simulink model "Table_de_mixage"  (R2020a)
settings: Solver=VariableStepAuto  StartTime=0.0  StopTime=10.0  RelTol=1e-3
undefined symbols (not defined in the file): fdesignblkfcn, gcbh
libraries: dspspect3 x3, dsparch4 x1, dspsrcs4 x1, dspvision x1, dspobslib x1, simulink x1
settings Model: Creator=XPS 15  LastModifiedBy=XPS 15

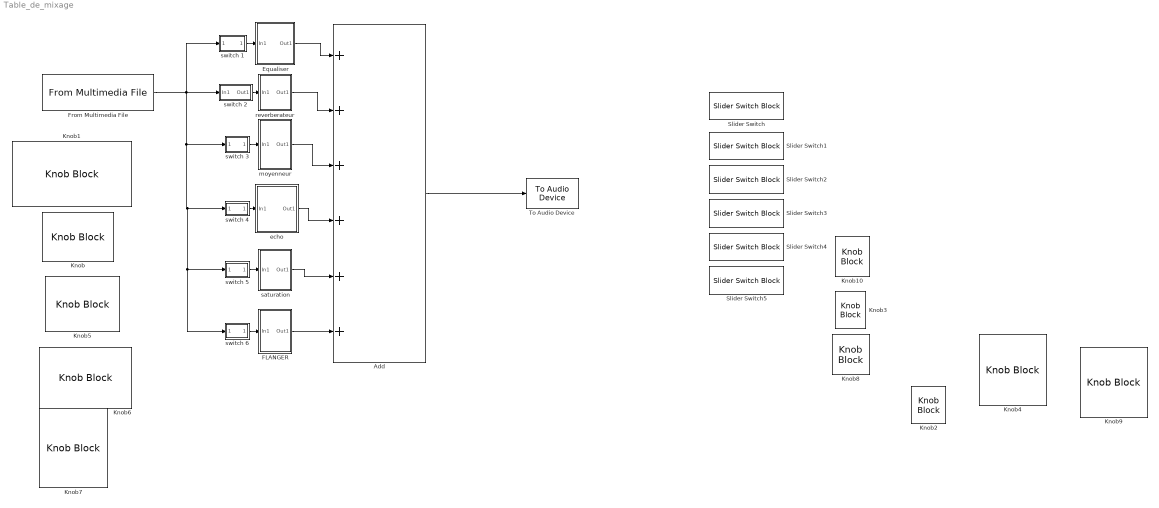
== system Table_de_mixage ==
  Add : Sum  Inputs=++++++
  Equaliser : Subsystem
  FLANGER : Subsystem
  From Multimedia File : dspvision/From Multimedia File  inputFilename=C:\Users\XPS 15\Desktop\L05 Sorbonne\images\Son\Projet\guitare.wav  readRange=[1 Inf]  loop=on  numPlays=inf  outputStreams=Audio only  videoDataType=single  audioDataType=double  inheritSampleTime=on  userDefinedSampleTime=1/30  noAudioOutput=off  isIntensityVideo=off  fourcc=RGB  colorVideoFormat=Separate color signals  outputEOF=off  dataOrg=Column-major  audioFrameSize=11025  computeAudioFrameSize=off  outSamplingMode=Sample based
  Knob{,1,3,5..8,10} (8 alike) : KnobBlock  ScaleMax=1
  Knob2 : KnobBlock
  Knob4 : KnobBlock
  Knob9 : KnobBlock
  Slider Switch{,1..5} (6 alike) : SliderSwitchBlock
      settings: Values={{'Off', 'On'}, [0 1]}
  To Audio Device : dspobslib/To Audio Device  deviceName=Default  inheritSampleRate=on  sampleRate=44100  deviceDatatype=Determine from input data type  autoBufferSize=on  bufferSize=4096  queueDuration=1.0  defaultOutputChannelMapping=on  outputChannelMapping=1:2  outputNumUnderrunSamples=off
      settings: SourceProductBaseCode=DS
  echo : Subsystem
  moyenneur : Subsystem
  reverberateur : Subsystem
  saturation : Subsystem
  switch 1 : Subsystem
  switch 2 : Subsystem
  switch 3 : Subsystem
  switch 4 : Subsystem
  switch 5 : Subsystem
  switch 6 : Subsystem
  wires:
  Equaliser/1(Out1) -> Add/1
  saturation/1(Out1) -> Add/5
  echo/1(Out1) -> Add/4
  moyenneur/1(Out1) -> Add/3
  reverberateur/1(Out1) -> Add/2
  switch 1/1(Out1) -> Equaliser/1(In1)
  From Multimedia File/1 -> switch 6/1(In1), switch 5/1(In1), switch 4/1(In1), switch 3/1(In1), switch 2/1(In1), switch 1/1(In1)
  switch 2/1(Out1) -> reverberateur/1(In1)
  switch 3/1(Out1) -> moyenneur/1(In1)
  switch 4/1(Out1) -> echo/1(In1)
  switch 5/1(Out1) -> saturation/1(In1)
  FLANGER/1(Out1) -> Add/6
  switch 6/1(Out1) -> FLANGER/1(In1)
  Add/1 -> To Audio Device/1

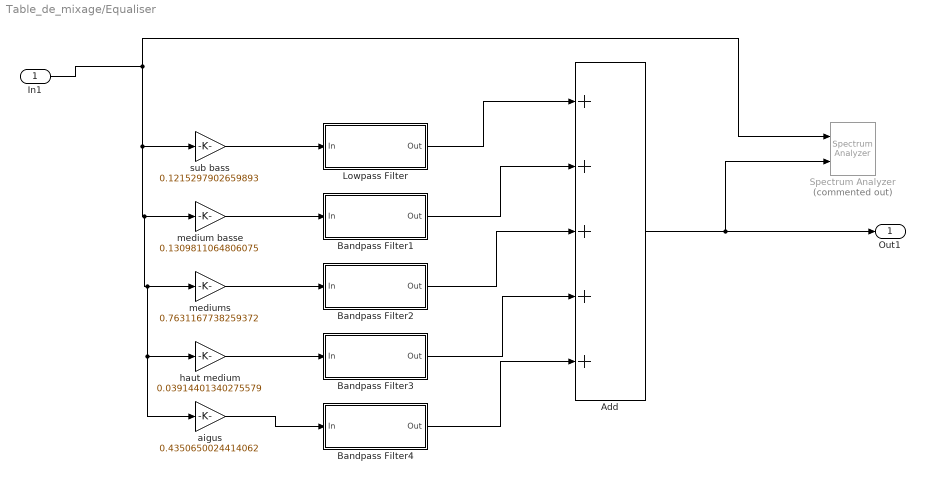
== system Table_de_mixage/Equaliser ==
  In1 : Inport
  Add : Sum  Inputs=+++++
  Bandpass Filter1 : Subsystem  DialogController=fdesignblkfcn  InitFcn=fdesignblkfcn(gcbh, {'InitFcn'});  mask(Bandpass Filter){}
      mask help: Design a bandpass filter
      settings: CopyFcn=fdesignblkfcn(gcbh, {'CopyFcn'});
      mask Help: helpview(mapfilelocation('dsp'), 'dspbandpassfilter');
      mask Display: disp('Bandpass');
  Bandpass Filter2 : Subsystem  DialogController=fdesignblkfcn  InitFcn=fdesignblkfcn(gcbh, {'InitFcn'});  mask(Bandpass Filter){}
      mask help: Design a bandpass filter
      settings: CopyFcn=fdesignblkfcn(gcbh, {'CopyFcn'});
      mask Help: helpview(mapfilelocation('dsp'), 'dspbandpassfilter');
      mask Display: disp('Bandpass');
  Bandpass Filter3 : Subsystem  DialogController=fdesignblkfcn  InitFcn=fdesignblkfcn(gcbh, {'InitFcn'});  mask(Bandpass Filter){}
      mask help: Design a bandpass filter
      settings: CopyFcn=fdesignblkfcn(gcbh, {'CopyFcn'});
      mask Help: helpview(mapfilelocation('dsp'), 'dspbandpassfilter');
      mask Display: disp('Bandpass');
  Bandpass Filter4 : Subsystem  DialogController=fdesignblkfcn  InitFcn=fdesignblkfcn(gcbh, {'InitFcn'});  mask(Bandpass Filter){}
      mask help: Design a bandpass filter
      settings: CopyFcn=fdesignblkfcn(gcbh, {'CopyFcn'});
      mask Help: helpview(mapfilelocation('dsp'), 'dspbandpassfilter');
      mask Display: disp('Bandpass');
  Lowpass Filter : Subsystem  DialogController=fdesignblkfcn  InitFcn=fdesignblkfcn(gcbh, {'InitFcn'});  mask(Lowpass Filter){}
      mask help: Design a lowpass filter
      settings: CopyFcn=fdesignblkfcn(gcbh, {'CopyFcn'});
      mask Help: helpview(mapfilelocation('dsp'), 'dsplowpassfilter');
      mask Display: disp('Lowpass')
  Spectrum Analyzer : SpectrumAnalyzer  Commented=on  NumInputPorts=2
  aigus : Gain  Gain=0.4350650024414062
  haut medium : Gain  Gain=0.03914401340275579
  medium basse : Gain  Gain=0.1309811064806075
  mediums : Gain  Gain=0.7631167738259372
  sub bass : Gain  Gain=0.1215297902659893
  Out1 : Outport
  wires:
  Lowpass Filter/1(Out) -> Add/1
  haut medium/1 -> Bandpass Filter3/1(In)
  sub bass/1 -> Lowpass Filter/1(In)
  In1/1 -> aigus/1, haut medium/1, mediums/1, medium basse/1, sub bass/1, Spectrum Analyzer/1
  mediums/1 -> Bandpass Filter2/1(In)
  Bandpass Filter3/1(Out) -> Add/4
  Add/1 -> Out1/1, Spectrum Analyzer/2
  medium basse/1 -> Bandpass Filter1/1(In)
  Bandpass Filter2/1(Out) -> Add/3
  Bandpass Filter4/1(Out) -> Add/5
  aigus/1 -> Bandpass Filter4/1(In)
  Bandpass Filter1/1(Out) -> Add/2

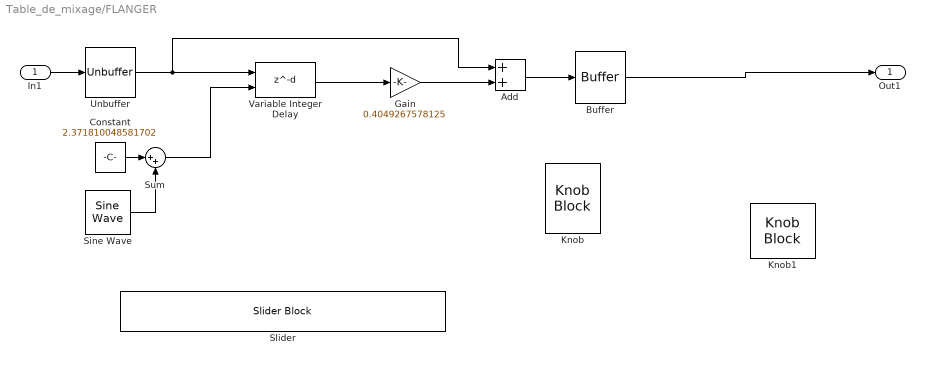
== system Table_de_mixage/FLANGER ==
  In1 : Inport
  Add : Sum
  Buffer : Buffer  N=11025  OutputFrames=off
  Constant : Constant  Value=2.371810048581702
  Gain : Gain  Gain=0.4049267578125
  Knob : KnobBlock  ScaleMax=5
  Knob1 : KnobBlock  ScaleMax=1
  Sine Wave : dspsrcs4/Sine Wave  Amplitude=1  Frequency=804.9368351063829  Phase=0  SampleMode=Discrete  OutComplex=Real  CompMethod=Trigonometric fcn  TableSize=Speed  SampleTime=1/11025  SamplesPerFrame=1  ResetState=Restart at time zero  OutputFrames=off  dataType=double  wordLen=16  udDataType=sfix(16)  fracBitsMode=Best precision  numFracBits=15  OutDataTypeStr=double  LastOutDataTypeStr=double
  Slider : SliderBlock  ScaleMax=10000
  Sum : Sum  Inputs=|++
  Unbuffer : Unbuffer
  Variable Integer Delay : Delay  DelayLengthSource=Input port
      settings: InputPortMap=u0,p1
  Out1 : Outport
  wires:
  In1/1 -> Unbuffer/1
  Unbuffer/1 -> Add/1, Variable Integer Delay/1
  Constant/1 -> Sum/1
  Sine Wave/1 -> Sum/2
  Sum/1 -> Variable Integer Delay/2
  Variable Integer Delay/1 -> Gain/1
  Gain/1 -> Add/2
  Add/1 -> Buffer/1
  Buffer/1 -> Out1/1

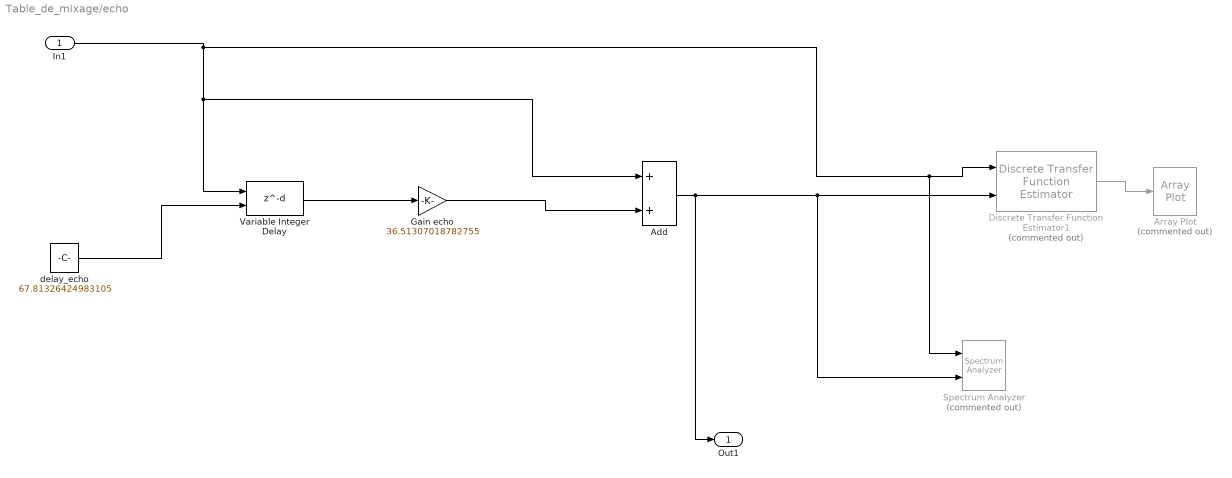
== system Table_de_mixage/echo ==
  In1 : Inport
  Add : Sum
  Array Plot : ArrayPlot  Commented=on
  Discrete Transfer Function Estimator1 : dspspect3/Discrete Transfer Function Estimator  Commented=on  WindowMode=Specify on dialog  WindowLength=1024  Overlap=50  AveragingMethod=Running  ForgettingFactorPort=off  ForgettingFactor=0.9  SpectralAverages=100  FFTLengthSource=Auto  FFTLength=128  Window=Hann  SidelobeAttenuation=60  FrequencyRange=One-sided  OutputCoherence=off  SimulateUsing=Code generation
      settings: SourceProductBaseCode=DS
  Gain echo : Gain  Gain=36.51307018782755
  Spectrum Analyzer : SpectrumAnalyzer  Commented=on  NumInputPorts=2
  Variable Integer Delay : Delay  DelayLengthSource=Input port
      settings: InputPortMap=u0,p1
  delay_echo : Constant  Value=67.81326424983105
  Out1 : Outport
  wires:
  Add/1 -> Discrete Transfer Function Estimator1/2, Spectrum Analyzer/2, Out1/1
  Variable Integer Delay/1 -> Gain echo/1
  In1/1 -> Variable Integer Delay/1, Add/1, Spectrum Analyzer/1, Discrete Transfer Function Estimator1/1
  Gain echo/1 -> Add/2
  Discrete Transfer Function Estimator1/1 -> Array Plot/1
  delay_echo/1 -> Variable Integer Delay/2

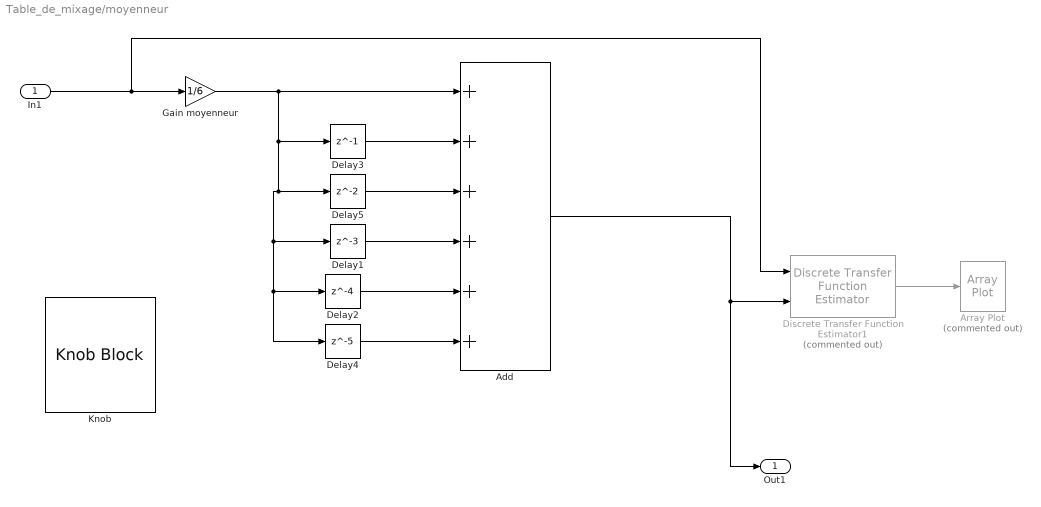
== system Table_de_mixage/moyenneur ==
  In1 : Inport
  Add : Sum  Inputs=++++++
  Array Plot : ArrayPlot  Commented=on
  Delay1 : Delay  DelayLength=3  InitialCondition=0  InputProcessing=Columns as channels (frame based)
  Delay2 : Delay  DelayLength=4  InitialCondition=0  InputProcessing=Columns as channels (frame based)
  Delay3 : Delay  DelayLength=1  InitialCondition=0  InputProcessing=Columns as channels (frame based)
  Delay4 : Delay  DelayLength=5  InitialCondition=0  InputProcessing=Columns as channels (frame based)
  Delay5 : Delay  InitialCondition=0  InputProcessing=Columns as channels (frame based)
  Discrete Transfer Function Estimator1 : dspspect3/Discrete Transfer Function Estimator  Commented=on  WindowMode=Specify on dialog  WindowLength=1024  Overlap=50  AveragingMethod=Running  ForgettingFactorPort=off  ForgettingFactor=0.9  SpectralAverages=100  FFTLengthSource=Auto  FFTLength=128  Window=Hann  SidelobeAttenuation=60  FrequencyRange=One-sided  OutputCoherence=off  SimulateUsing=Code generation
      settings: SourceProductBaseCode=DS
  Gain moyenneur : Gain  Gain=1/6
  Knob : KnobBlock
  Out1 : Outport
  wires:
  Delay4/1 -> Add/6
  Delay5/1 -> Add/3
  Gain moyenneur/1 -> Delay5/1, Delay1/1, Delay2/1, Delay4/1, Delay3/1, Add/1
  Discrete Transfer Function Estimator1/1 -> Array Plot/1
  Delay1/1 -> Add/4
  Add/1 -> Out1/1, Discrete Transfer Function Estimator1/2
  Delay2/1 -> Add/5
  In1/1 -> Discrete Transfer Function Estimator1/1, Gain moyenneur/1
  Delay3/1 -> Add/2

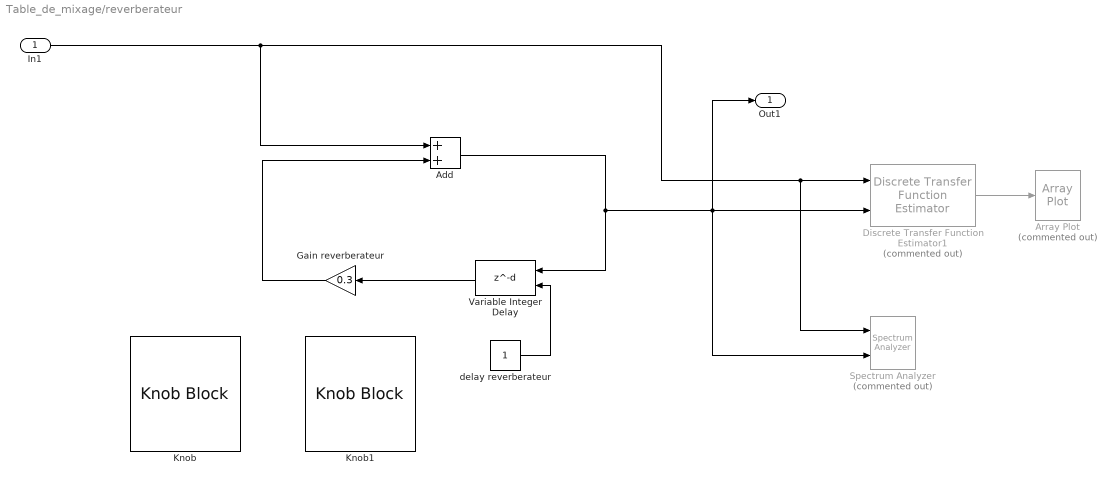
== system Table_de_mixage/reverberateur ==
  In1 : Inport
  Add : Sum
  Array Plot : ArrayPlot  Commented=on
  Discrete Transfer Function Estimator1 : dspspect3/Discrete Transfer Function Estimator  Commented=on  WindowMode=Specify on dialog  WindowLength=1024  Overlap=50  AveragingMethod=Running  ForgettingFactorPort=off  ForgettingFactor=0.9  SpectralAverages=100  FFTLengthSource=Auto  FFTLength=128  Window=Hann  SidelobeAttenuation=60  FrequencyRange=One-sided  OutputCoherence=off  SimulateUsing=Code generation
      settings: SourceProductBaseCode=DS
  Gain reverberateur : Gain  Gain=0.3
  Knob : KnobBlock
  Knob1 : KnobBlock
  Spectrum Analyzer : SpectrumAnalyzer  Commented=on  NumInputPorts=2
  Variable Integer Delay : Delay  DelayLengthSource=Input port
      settings: InputPortMap=u0,p1
  delay reverberateur : Constant
  Out1 : Outport
  wires:
  Discrete Transfer Function Estimator1/1 -> Array Plot/1
  Gain reverberateur/1 -> Add/2
  Variable Integer Delay/1 -> Gain reverberateur/1
  In1/1 -> Spectrum Analyzer/1, Discrete Transfer Function Estimator1/1, Add/1
  Add/1 -> Variable Integer Delay/1, Out1/1, Spectrum Analyzer/2, Discrete Transfer Function Estimator1/2
  delay reverberateur/1 -> Variable Integer Delay/2

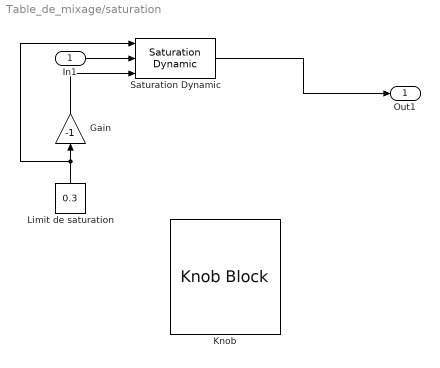
== system Table_de_mixage/saturation ==
  In1 : Inport
  Gain : Gain  Gain=-1
  Knob : KnobBlock
  Limit de saturation : Constant  Value=0.3
  Saturation Dynamic : simulink/Discontinuities/Saturation Dynamic  OutMin=[]  OutMax=[]  OutDataTypeStr=Inherit: Same as second input  OutDataType=fixdt(1, 16)  OutScaling=2^-10  DoSatur=off
  Out1 : Outport
  wires:
  Limit de saturation/1 -> Saturation Dynamic/1, Gain/1
  Gain/1 -> Saturation Dynamic/3
  In1/1 -> Saturation Dynamic/2
  Saturation Dynamic/1 -> Out1/1

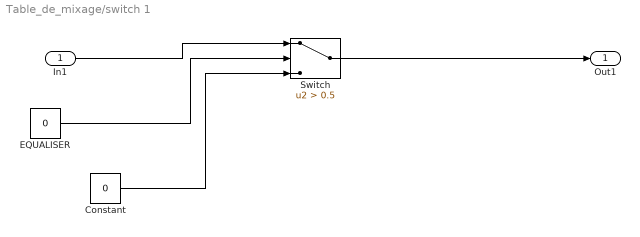
== system Table_de_mixage/switch 1 ==
  In1 : Inport
  Constant : Constant  Value=0
  EQUALISER : Constant  Value=0
  Switch : Switch  Criteria=u2 > Threshold  Threshold=0.5
  Out1 : Outport
  wires:
  EQUALISER/1 -> Switch/2
  Constant/1 -> Switch/3
  Switch/1 -> Out1/1
  In1/1 -> Switch/1

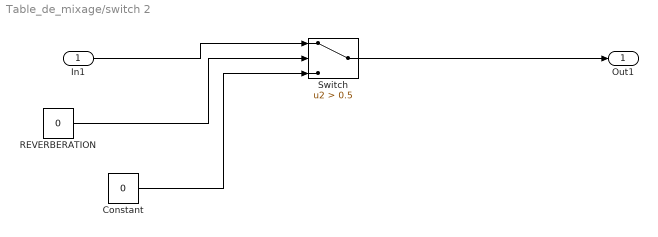
== system Table_de_mixage/switch 2 ==
  In1 : Inport
  Constant : Constant  Value=0
  REVERBERATION : Constant  Value=0
  Switch : Switch  Criteria=u2 > Threshold  Threshold=0.5
  Out1 : Outport
  wires:
  In1/1 -> Switch/1
  Switch/1 -> Out1/1
  Constant/1 -> Switch/3
  REVERBERATION/1 -> Switch/2

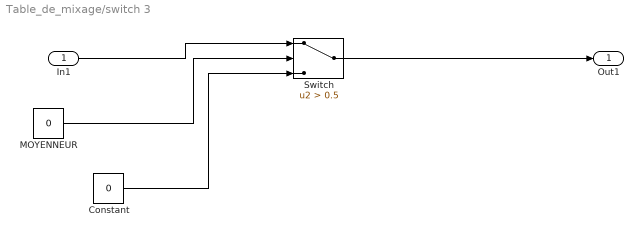
== system Table_de_mixage/switch 3 ==
  In1 : Inport
  Constant : Constant  Value=0
  MOYENNEUR : Constant  Value=0
  Switch : Switch  Criteria=u2 > Threshold  Threshold=0.5
  Out1 : Outport
  wires:
  MOYENNEUR/1 -> Switch/2
  Constant/1 -> Switch/3
  Switch/1 -> Out1/1
  In1/1 -> Switch/1

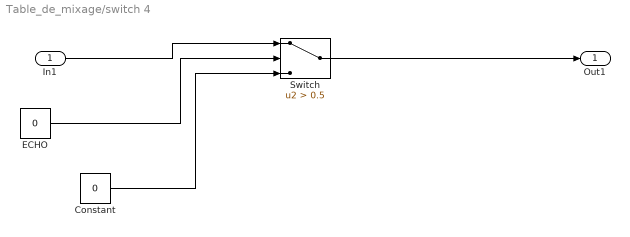
== system Table_de_mixage/switch 4 ==
  In1 : Inport
  Constant : Constant  Value=0
  ECHO : Constant  Value=0
  Switch : Switch  Criteria=u2 > Threshold  Threshold=0.5
  Out1 : Outport
  wires:
  ECHO/1 -> Switch/2
  Constant/1 -> Switch/3
  Switch/1 -> Out1/1
  In1/1 -> Switch/1

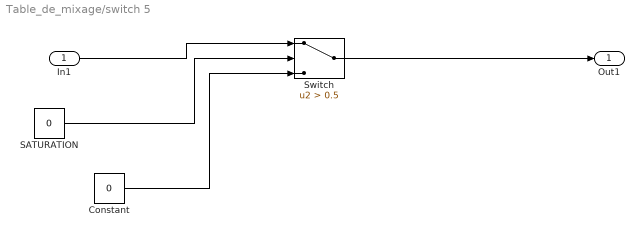
== system Table_de_mixage/switch 5 ==
  In1 : Inport
  Constant : Constant  Value=0
  SATURATION : Constant  Value=0
  Switch : Switch  Criteria=u2 > Threshold  Threshold=0.5
  Out1 : Outport
  wires:
  SATURATION/1 -> Switch/2
  Constant/1 -> Switch/3
  Switch/1 -> Out1/1
  In1/1 -> Switch/1

== system Table_de_mixage/switch 6 ==
  In1 : Inport
  Constant : Constant  Value=0
  FLANGER : Constant
  Switch : Switch  Criteria=u2 > Threshold  Threshold=0.5
  Out1 : Outport
  wires:
  In1/1 -> Switch/1
  Switch/1 -> Out1/1
  Constant/1 -> Switch/3
  FLANGER/1 -> Switch/2

== system Table_de_mixage/Equaliser/Bandpass Filter1 ==
  In : Inport
  Generated Filter Block : DiscreteFir  Tag=BlockMethodSubSystem  Coefficients=[-0.243892203726465723 0.00730478846362643628 0.00727026155694758622 0.0072195879313937273 0.00718013595561857107 0.00712564556376517333 0.00715711381682971205 0.00714005369985488275 0.00721758291259837551 0.00723368155872983979 0.00734625490622398559 0.00739114557287962916 0.00753271554443431593 0.00760297693046721717 0.00776943129724880048 0.00786214348435359915 0.00805013251467046748 0.00816254346016220649 0.00836893604947036227 0.00849825547017768121 0.00871982829709244157 0.00886309417338047335 0.00909628249041599321 0.00925025614094075223 0.00949081341540646169 0.00965184580644971521 0.00989406171868761029 0.0100577734886275576 0.0102918492194648513 0.0104519182300895179 0.0106506090885365758 0.0107916127474229177 0.0107424423140313665 0.01144347505709567 0.0115420964215233318 0.0116650592912086876 0.011681173358027765 0.0117975571295101892 0.0119616385119765394 0.0120692530210493257 0.0122409746268588356 0.0123291328786560937 0.0124866423972848639 0.0125508784741977849 0.0126863271368207239 0.0127238269503861107 0.0128331605186119881 0.0128420197478149017 0.0129228716119024964 0.0129019498716525152 0.0129530389564096599 0.0129019498716525152 0.0129228716119024964 0.0128420197478149017 0.0128331605186119881 0.0127238269503861107 0.0126863271368207239 0.0125508784741977849 0.0124866423972848639 0.0123291328786560937 0.0122409746268588356 0.0120692530210493257 0.0119616385119765394 0.0117975571295101892 0.011681173358027765 0.0116650592912086876 0.0115420964215233318 0.01144347505709567 0.0107424423140313665 0.0107916127474229177 0.0106506090885365758 0.0104519182300895179 0.0102918492194648513 0.0100577734886275576 0.00989406171868761029 0.00965184580644971521 0.00949081341540646169 0.00925025614094075223 0.00909628249041599321 0.00886309417338047335 0.00871982829709244157 0.00849825547017768121 0.00836893604947036227 0.00816254346016220649 0.00805013251467046748 0.00786214348435359915 0.00776943129724880048 0.00760297693046721717 0.00753271554443431593 0.00739114557287962916 0.00734625490622398559 0.00723368155872983979 0.00721758291259837551 0.00714005369985488275 0.00715711381682971205 0.00712564556376517333 0.00718013595561857107 0.0072195879313937273 0.00727026155694758622 0.00730478846362643628 -0.243892203726465723]  InputProcessing=Columns as channels (frame based)
  Out : Outport
  wires:
  Generated Filter Block/1 -> Out/1
  In/1 -> Generated Filter Block/1

== system Table_de_mixage/Equaliser/Bandpass Filter2 ==
  In : Inport
  Generated Filter Block : DiscreteFir  Tag=BlockMethodSubSystem  Coefficients=[-0.219992515160361196 0.00041067924301887613 -0.000955230595402657137 -0.00316298935289945115 -0.00580833419451566319 -0.00875259525417781264 -0.0116667781153422696 -0.0141526454179858804 -0.0158994316506139675 -0.0166510425615134169 -0.0160921844465764553 -0.0140581982025706417 -0.0105091030386617566 -0.0053635112224876191 0.00132332363263672334 0.00917842095473490709 0.0180397330213489561 0.027888794657402783 0.0374895690389822692 0.0468915263196734364 0.0562236340265577922 0.0641391808900700217 0.070902870795508971 0.0758376849051398821 0.0790158094717990228 0.0799663131981928205 0.0790158094717990228 0.0758376849051398821 0.070902870795508971 0.0641391808900700217 0.0562236340265577922 0.0468915263196734364 0.0374895690389822692 0.027888794657402783 0.0180397330213489561 0.00917842095473490709 0.00132332363263672334 -0.0053635112224876191 -0.0105091030386617566 -0.0140581982025706417 -0.0160921844465764553 -0.0166510425615134169 -0.0158994316506139675 -0.0141526454179858804 -0.0116667781153422696 -0.00875259525417781264 -0.00580833419451566319 -0.00316298935289945115 -0.000955230595402657137 0.00041067924301887613 -0.219992515160361196]  InputProcessing=Columns as channels (frame based)
  Out : Outport
  wires:
  Generated Filter Block/1 -> Out/1
  In/1 -> Generated Filter Block/1

== system Table_de_mixage/Equaliser/Bandpass Filter3 ==
  In : Inport
  Generated Filter Block : DiscreteFir  Tag=BlockMethodSubSystem  Coefficients=[-0.0574675757817210767 0.0328729305641321523 0.0153181963810936576 0.0144000921568288899 0.0271562000272343555 0.0367681084965816307 0.0305362503447960572 0.0130025466067944153 0.00138953688409791318 0.00704909955959066772 0.0233811928243845522 0.0307456244346326173 0.0152933718616004456 -0.0156791567588090187 -0.0391235456259758224 -0.0365287210407774024 -0.0130684100901103939 0.00344522185635996389 -0.0145546538735224652 -0.0676940657813424607 -0.121272411524454574 -0.126465671108468986 -0.0562876428509682669 0.0689920044301164936 0.188699491423545251 0.237826339431704836 0.188699491423545251 0.0689920044301164936 -0.0562876428509682669 -0.126465671108468986 -0.121272411524454574 -0.0676940657813424607 -0.0145546538735224652 0.00344522185635996389 -0.0130684100901103939 -0.0365287210407774024 -0.0391235456259758224 -0.0156791567588090187 0.0152933718616004456 0.0307456244346326173 0.0233811928243845522 0.00704909955959066772 0.00138953688409791318 0.0130025466067944153 0.0305362503447960572 0.0367681084965816307 0.0271562000272343555 0.0144000921568288899 0.0153181963810936576 0.0328729305641321523 -0.0574675757817210767]  InputProcessing=Columns as channels (frame based)
  Out : Outport
  wires:
  Generated Filter Block/1 -> Out/1
  In/1 -> Generated Filter Block/1

== system Table_de_mixage/Equaliser/Bandpass Filter4 ==
  In : Inport
  Generated Filter Block : DiscreteFir  Tag=BlockMethodSubSystem  Coefficients=[-0.00250578981709462289 -0.0442617374483873921 0.0520018635513649352 0.002449797309117022 -0.0245881630666010612 -0.0394709414897238403 -0.0435778581430307441 -0.0382951499420577171 -0.0248693538842632601 -0.00547565673543737655 0.0162839773169923506 0.0356451905802601596 0.0477574698504968712 0.0487545944562484887 0.0372470431594712839 0.0150148458334138004 -0.0128177527641289875 -0.0394966613630594529 -0.0579387995789589633 -0.0624675285538587588 -0.0515422534389315193 -0.027035034064764759 0.00499660823923454324 0.0366073935269759648 0.0595530085754514549 0.0679508762259099369 0.0595530085754514549 0.0366073935269759648 0.00499660823923454324 -0.027035034064764759 -0.0515422534389315193 -0.0624675285538587588 -0.0579387995789589633 -0.0394966613630594529 -0.0128177527641289875 0.0150148458334138004 0.0372470431594712839 0.0487545944562484887 0.0477574698504968712 0.0356451905802601596 0.0162839773169923506 -0.00547565673543737655 -0.0248693538842632601 -0.0382951499420577171 -0.0435778581430307441 -0.0394709414897238403 -0.0245881630666010612 0.002449797309117022 0.0520018635513649352 -0.0442617374483873921 -0.00250578981709462289]  InputProcessing=Columns as channels (frame based)
  Out : Outport
  wires:
  Generated Filter Block/1 -> Out/1
  In/1 -> Generated Filter Block/1

== system Table_de_mixage/Equaliser/Lowpass Filter ==
  In : Inport
  Generated Filter Block : dsparch4/Biquad Filter  Tag=BlockMethodSubSystem  FilterSource=Dialog parameters  CoeffSource=Specify via dialog  FilterObject=BQF  IIRFiltStruct=Direct form II  BiQuadCoeffs=[0.0563723868047192808 -0.112733102282839351 0.0563723868047192669 1 -1.99986709090954307 0.999938785053186452;0.134974380184157555 -0.269917274952083008 0.134974380184157527 1 -1.99977389867106825 0.999837538604667841;0.173920984013434643 -0.347789697719413093 0.173920984013434615 1 -1.99968088212988682 0.999730294111489282;0.142800419806492385 -0.285533255599871194 0.142800419806492357 1 -1.99959043502248424 0.999621839640458254;0.0505605581933390794 -0.101066832109269797 0.0505605581933390655 1 -1.99951302399492192 0.9995269074452372;0.000106461863219572045 -0.000212210004753128612 0.000106461863219572031 1 -1.99946472971333922 0.999467012303375313;4.40883755804437889e-05 -8.11633175447999255e-05 4.40883755804437821e-05 1 -1.99945608647293382 0.999456250056217632;0.0104168059304009155 -0.0208113611700088477 0.0104168059304009172 1 -1.99948421122565123 0.999491224659267319;0.0608092620572879133 -0.121577866165242549 0.0608092620572879133 1 -1.99954915400870048 0.999571404699493571;0.156525699636279131 -0.312994209691630887 0.156525699636279131 1 -1.99963487361091174 0.999675531560245134;0.263947331311924993 -0.527826138170822912 0.263947331311925049 1 -1.99972739768301588 0.999784587263943147;0.337297340504941146 -0.674521614069119035 0.33729734050494109 1 -1.99982034766155059 0.999888872114577665;0.0136480036810581167 -0.0272932347749923442 0.013648003681058115 1 -1.99991473696685018 0.999987803907613326;0.076461893140403997 -0.152907648374149358 0.0764618931404039831 1 -1.9998436491163436 0.999913979229615779;0.150508444553466902 -0.300980015464457296 0.150508444553466875 1 -1.99975066265285961 0.999811260610833141;0.172623556004974726 -0.34519030126451461 0.172623556004974699 1 -1.99965776099161596 0.999702891213229861;0.112565860401863796 -0.225069206516408188 0.112565860401863838 1 -1.9995692825564455 0.999596056297053615;0.00516349076946631593 -0.0103194354849358589 0.0051634907694663142 1 -1.99949756929435418 0.999507787658860281;0.000228414384351603901 -0.000452625013012197559 0.000228414384351603955 1 -1.99945898779652342 0.99945986399859299;0.00512541605497199466 -0.0102330536537159032 0.00512541605497199727 1 -1.99947319401283607 0.999477539987490782;0.0432407703237225258 -0.0864456221816943676 0.0432407703237225188 1 -1.99953031031732875 0.999548234210902109;0.129396534304628413 -0.258739748926119784 0.129396534304628441 1 -1.99961237030849204 0.999648429204505917;0.237053760705792482 -0.474041664133251217 0.237053760705792538 1 -1.99970412142491294 0.999757569047541095;0.229454335606285337 -0.458857287834215644 0.229454335606285281 1 -1.99979711565747698 0.999863404709366299;1.00010222666177384 -2 1.00010222666177362 1 -1.999890756337102 0.999963364523810072]  ScaleValues=[7.29746110296593831e-07;1;1;1;1;1;1;1;1;1;1;1;1;1;1;1;1;1;1;1;1;1;1;1;1;6781.3111062025182]  IC=0  ICnum=0  ICden=0  a0Flag=Warning  optimizeScaleValues=off  ScaleValueMode=Specify via input port (g)  InputProcessing=Columns as channels (frame based)  roundingMode=Floor  overflowMode=off  scaleValueFracLength=14  denProdOutputFracLength=30  denAccumFracLength=30  secondMemoryFracLength=15
  Out : Outport
  wires:
  Generated Filter Block/1 -> Out/1
  In/1 -> Generated Filter Block/1
